simulink model "debris_model"  (R2016a)
settings: Solver=VariableStepAuto  StartTime=0.0  StopTime=10.0  RelTol=1e-3
values from neighbouring files (symbols this model uses):
  DBG = [MB.m*eye(3) zeros(3,3);zeros(3,3) MB.I]    [exemple_debris.m]    (also in sat_dynamics.m)
  SA_Dyn = ss(aa,bb,cc,dd)    [exemple_debris.m]
  SCtauCGP = [eye(3) -[0 CGPvec(3) -CGPvec(2) ... (first row only)    [exemple_debris.m]    (also in sat_dynamics.m)
undefined symbols (not defined in the file or in its folder): minreal, SA
libraries: cstblocks x3
settings Model: Creator=f.sanfedino  LastModifiedBy=f.sanfedino

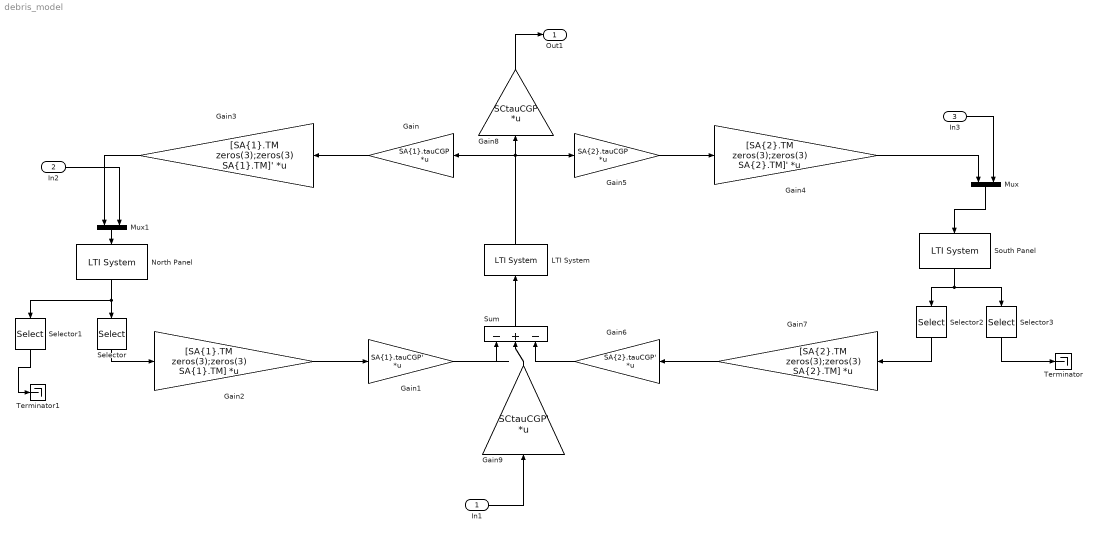
== system debris_model ==
  In1 : Inport  PortDimensions=6
  In2 : Inport  Port=2  PortDimensions=6
  In3 : Inport  Port=3  PortDimensions=6
  Gain : Gain  Gain=SA{1}.tauCGP  Multiplication=Matrix(K*u)
  Gain1 : Gain  Gain=SA{1}.tauCGP'  Multiplication=Matrix(K*u)
  Gain2 : Gain  Gain=[SA{1}.TM zeros(3);zeros(3) SA{1}.TM]  Multiplication=Matrix(K*u)
  Gain3 : Gain  Gain=[SA{1}.TM zeros(3);zeros(3) SA{1}.TM]'  Multiplication=Matrix(K*u)
  Gain4 : Gain  Gain=[SA{2}.TM zeros(3);zeros(3) SA{2}.TM]'  Multiplication=Matrix(K*u)
  Gain5 : Gain  Gain=SA{2}.tauCGP  Multiplication=Matrix(K*u)
  Gain6 : Gain  Gain=SA{2}.tauCGP'  Multiplication=Matrix(K*u)
  Gain7 : Gain  Gain=[SA{2}.TM zeros(3);zeros(3) SA{2}.TM]  Multiplication=Matrix(K*u)
  Gain8 : Gain  Gain=SCtauCGP  Multiplication=Matrix(K*u)
  Gain9 : Gain  Gain=SCtauCGP'  Multiplication=Matrix(K*u)
  LTI System : cstblocks/LTI System  sys=inv(DBG)  IC=[]
  Mux : Mux  Inputs=2
  Mux1 : Mux  Inputs=2
  North Panel : cstblocks/LTI System  sys=minreal(SA_Dyn)  IC=[]
  Selector : Selector  InputPortWidth=12  IndexOptions=Index vector (dialog)  Indices=[1:6]  OutputSizes=1
  Selector1 : Selector  InputPortWidth=12  IndexOptions=Index vector (dialog)  Indices=[7:12]  OutputSizes=1
  Selector2 : Selector  InputPortWidth=12  IndexOptions=Index vector (dialog)  Indices=[1:6]  OutputSizes=1
  Selector3 : Selector  InputPortWidth=12  IndexOptions=Index vector (dialog)  Indices=[7:12]  OutputSizes=1
  South Panel : cstblocks/LTI System  sys=minreal(SA_Dyn)  IC=[]
  Sum : Sum  Inputs=|-+-
  Terminator : Terminator
  Terminator1 : Terminator
  Out1 : Outport
  wires:
  Gain2/1 -> Gain1/1
  Gain/1 -> Gain3/1
  Gain3/1 -> Mux1/1
  Selector/1 -> Gain2/1
  LTI System/1 -> Gain/1, Gain8/1, Gain5/1
  Sum/1 -> LTI System/1
  Gain1/1 -> Sum/1
  Gain5/1 -> Gain4/1
  Gain6/1 -> Sum/3
  Gain7/1 -> Gain6/1
  Gain4/1 -> Mux/1
  Selector2/1 -> Gain7/1
  Mux/1 -> South Panel/1
  Mux1/1 -> North Panel/1
  North Panel/1 -> Selector1/1, Selector/1
  South Panel/1 -> Selector3/1, Selector2/1
  In1/1 -> Gain9/1
  Selector3/1 -> Terminator/1
  Gain9/1 -> Sum/2
  In2/1 -> Mux1/2
  Gain8/1 -> Out1/1
  Selector1/1 -> Terminator1/1
  In3/1 -> Mux/2
